simulink model "EPD629_WilliamsJ_AS04_P4_simulink"  (R2021b)
settings: Solver=VariableStepAuto  StartTime=0.0  StopTime=1  RelTol=1e-3
values from neighbouring files (symbols this model uses):
  ArmatureVoltage = 10    [EPD629_WilliamsJ_AS04.m]
  b = 0.001    [EPD629_WilliamsJ_AS04.m]
  J = 50e-6    (= 5e-05)    [EPD629_WilliamsJ_AS04.m]
  K = 0.1    [EPD629_WilliamsJ_AS04.m]
  Kb = Kt    (= 0.063)    [EPD629_WilliamsJ_AS04.m]
  Kt = 0.063    [EPD629_WilliamsJ_AS04.m]
  L = 1e-3    (= 0.001)    [EPD629_WilliamsJ_AS04.m]
  R = 0.35    [EPD629_WilliamsJ_AS04.m]
undefined symbols (not defined in the file or in its folder): A4, B4, C4, D4
settings Model: Creator=jwilli42  LastModifiedBy=jwilli42

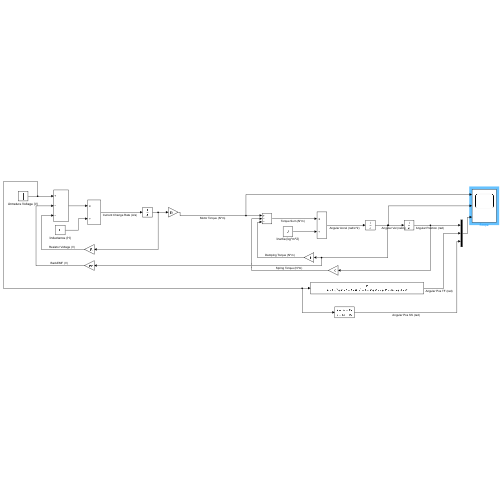
[thumbnail: Simulink's stored preview of the top-level diagram]
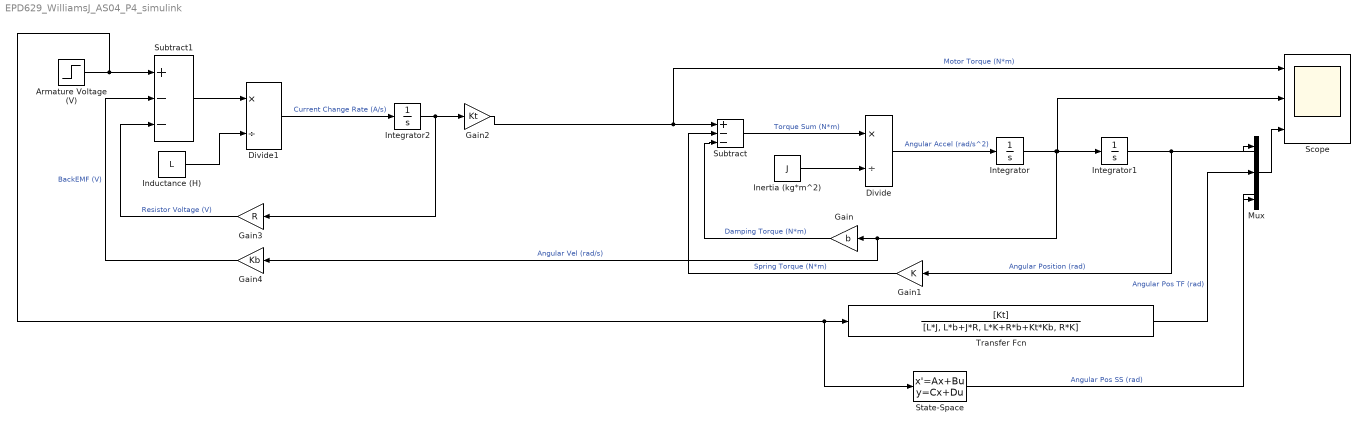
== system EPD629_WilliamsJ_AS04_P4_simulink ==
  Armature Voltage (V) : Step  Time=0  After=ArmatureVoltage  SampleTime=0
  Divide : Product  Inputs=*/
  Divide1 : Product  Inputs=*/
  Gain : Gain  Gain=b
  Gain1 : Gain  Gain=K
  Gain2 : Gain  Gain=Kt
  Gain3 : Gain  Gain=R
  Gain4 : Gain  Gain=Kb
  Inductance (H) : Constant  Value=L
  Inertia (kg*m^2) : Constant  Value=J
  Integrator : Integrator
  Integrator1 : Integrator
  Integrator2 : Integrator
  Mux : Mux  Inputs=3
  Scope : Scope  NumInputPorts=3
  State-Space : StateSpace  A=A4  B=B4  C=C4  D=D4  InitialCondition=0
  Subtract : Sum  Inputs=+--
  Subtract1 : Sum  Inputs=+--
  Transfer Fcn : TransferFcn  Numerator=[Kt]  Denominator=[L*J, L*b+J*R, L*K+R*b+Kt*Kb, R*K]
  wires:
  Gain2/1 -> Scope/1, Subtract/1  "Motor Torque (N*m)"
  Subtract/1 -> Divide/1  "Torque Sum (N*m)"
  Divide/1 -> Integrator/1  "Angular Accel (rad/s^2)"
  Integrator/1 -> Scope/2, Integrator1/1, Gain/1, Gain4/1  "Angular Vel (rad/s)"
  Inertia (kg*m^2)/1 -> Divide/2
  Gain/1 -> Subtract/3  "Damping Torque (N*m)"
  Mux/1 -> Scope/3
  Transfer Fcn/1 -> Mux/2  "Angular Pos TF (rad)"
  State-Space/1 -> Mux/3  "Angular Pos SS (rad)"
  Integrator1/1 -> Gain1/1, Mux/1  "Angular Position (rad)"
  Gain1/1 -> Subtract/2  "Spring Torque (N*m)"
  Armature Voltage (V)/1 -> Subtract1/1, State-Space/1, Transfer Fcn/1
  Subtract1/1 -> Divide1/1
  Inductance (H)/1 -> Divide1/2
  Divide1/1 -> Integrator2/1  "Current Change Rate (A/s)"
  Integrator2/1 -> Gain3/1, Gain2/1
  Gain3/1 -> Subtract1/3  "Resistor Voltage (V)"
  Gain4/1 -> Subtract1/2  "BackEMF (V)"
